simulink model "prova"  (R2023b)
settings: Solver=FixedStepAuto  StartTime=0.0  StopTime=100.0  RelTol=1e-3
settings Model: Creator=megan  LastModifiedBy=megan
settings OptimizationCC: DefaultParameterBehavior=Inlined  UseDivisionForNetSlopeComputation=on  GainParamInheritBuiltInType=on  UseFloatMulNetSlope=on  InlineInvariantSignals=on  EfficientFloat2IntCast=on  LifeSpan=1
settings HardwareCC: ProdLongLongMode=on
settings SFSimCC: MATLABDynamicMemAlloc=off
settings RTWCC: GenerateReport=on  LaunchReport=on
settings CodeAppCC: ForceParamTrailComments=on
settings GRTTargetCC: MatFileLogging=off

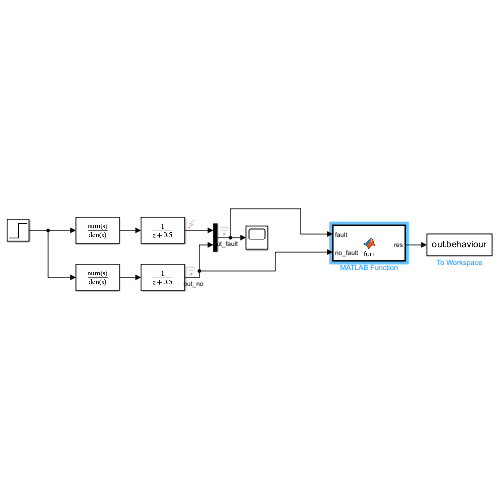
[thumbnail: Simulink's stored preview of the top-level diagram]
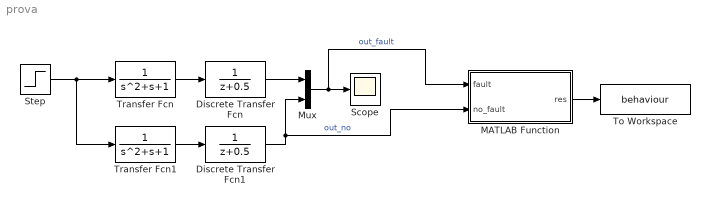
== system prova ==
  Discrete Transfer Fcn : DiscreteTransferFcn
  Discrete Transfer Fcn1 : DiscreteTransferFcn
  MATLAB Function : MATLAB Function  TreatAsAtomicUnit=on
  Mux : Mux  Inputs=2
  Scope : Scope
  Step : Step  SampleTime=0
  To Workspace : ToWorkspace  VariableName=behaviour  SaveFormat=Timeseries  SampleTime=-1
  Transfer Fcn : TransferFcn  Denominator=[1 1 1]
  Transfer Fcn1 : TransferFcn  Denominator=[1 1 1]
  wires:
  Discrete Transfer Fcn/1 -> Mux/1
  Mux/1 -> MATLAB Function/1(fault), Scope/1  "out_fault"
  Discrete Transfer Fcn1/1 -> MATLAB Function/2(no_fault), Mux/2  "out_no"
  Step/1 -> Transfer Fcn1/1, Transfer Fcn/1
  Transfer Fcn/1 -> Discrete Transfer Fcn/1
  Transfer Fcn1/1 -> Discrete Transfer Fcn1/1
  MATLAB Function/1(res) -> To Workspace/1

== matlab function prova/MATLAB Function ==
  data: fault input; no_fault input; res output
function res = fcn(fault, no_fault)

y = fault-no_fault;
res = isstable(y);
